simulink model "VCMGCM1962020b_v2"  (R2020b)
settings: Solver=FixedStepDiscrete  StartTime=0.0  StopTime=10.0  FixedStep=0.005  RelTol=1e-3  EnableMultiTasking=on
PreLoadFcn:
  | try, model_open; catch, disp('Error occurred while executing model pre-load callback: model_open.m'); disp('Please assure that the MATLAB working directory is set to the model directory before opening.'); end
InitFcn:
  | try, model_open; catch, end
undefined symbols (not defined in the file): Bridge, GCM, H, raptor_get_param_eval, raptor_get_safe_string, raptor_xcp_function
libraries: Blocks_lib x1165, Raptor_lib x665, simulink x62, VCM_lib x5
(part 17 of 23)

== system VCMGCM1962020b_v2/Fgnd/Control/Drive Inverter/Motor Torque Request/Inverter//Motor Limit & Request/Inverter Current Limit ==
  Split : Inport
  Bus Selector : BusSelector  OutputSignals=DrvInvtrMCLSplit [A],DrvInvtrGCLSplit [A]
  BusCreator : BusCreator  Inputs=2
  Header : Blocks_lib/Header  width=Portrait  addtext=''
  MinMax : MinMax  Inputs=2
  MinMax1 : MinMax  Inputs=2
  raptor_adjustment : Raptor_lib/Data Storage/raptor_adjustment  paramName=[invtrnam 'MCL']  nameSource=Parameter  initValue=0  dataType=double  storage=Calibration  calDispType=Number  calEnum={'Disabled', 'Enabled'}  calGain=1  calOffset=0  calMax=inf  calMin=-inf  calFormat=''  calUnit='A'  calHelp='Inverter motoring current limit'  calAccess=1  calFunction=group  calDispHeaders=off  calColHeaders={'Col1' 'Col2' 'Col3'}  calRowHeaders={'Row1' 'Row2' 'Row3'}
      settings: SourceProductName=Raptor
  raptor_adjustment1 : Raptor_lib/Data Storage/raptor_adjustment  paramName=[invtrnam 'GCL']  nameSource=Parameter  initValue=0  dataType=double  storage=Calibration  calDispType=Number  calEnum={'Disabled', 'Enabled'}  calGain=1  calOffset=0  calMax=inf  calMin=-inf  calFormat=''  calUnit='A'  calHelp='Inverter generating current limit'  calAccess=1  calFunction=group  calDispHeaders=off  calColHeaders={'Col1' 'Col2' 'Col3'}  calRowHeaders={'Row1' 'Row2' 'Row3'}
      settings: SourceProductName=Raptor
  InvtrCurLim : Outport  VectorParamsAs1DForOutWhenUnconnected=off
  wires:
  Bus Selector/1 -> MinMax/1  "<DrvInvtrMCLSplit [A]>"
  MinMax/1 -> BusCreator/1  "DrvInvtrMCL [A]"
  MinMax1/1 -> BusCreator/2  "DrvInvtrGCL [A]"
  BusCreator/1 -> InvtrCurLim/1  "InvtrCurLim"
  raptor_adjustment/1 -> MinMax/2
  raptor_adjustment1/1 -> MinMax1/2
  Split/1 -> Bus Selector/1
  Bus Selector/2 -> MinMax1/1  "<DrvInvtrGCLSplit [A]>"

== system VCMGCM1962020b_v2/Fgnd/Control/Drive Inverter/Motor Torque Request/Inverter//Motor Limit & Request/Motor Torque Limit ==
  Data : Inport
  EnblReq : Inport  Port=2
  InvtrCurLim : Inport  Port=3
  CAN : Subsystem
  Constant : Constant  Value=double([0 0])
  Current Control : Subsystem  mask{group=[group ' | Current Control']}
  Derate Multiplier : Subsystem
  Header : Blocks_lib/Header  width=Portrait  addtext=''
  Logical Operator : Logic  Operator=NOT  Inputs=1  AllPortsSameDT=off  OutDataTypeStr=boolean
  MinMax : MinMax  Inputs=3  InputSameDT=on
  MinMax1 : MinMax  Function=max  Inputs=3  InputSameDT=on
  Multiport Switch : MultiPortSwitch  DataPortOrder=Zero-based contiguous  Inputs=2  zeroidx=on
  Mux : Mux  Inputs=2
  Product : Product  InputSameDT=on  RndMeth=Zero  OutDataTypeStr=Inherit: Same as first input
  Product1 : Product  InputSameDT=on  RndMeth=Zero  OutDataTypeStr=Inherit: Same as first input
  Saturation : Saturate  UpperLimit=inf  LowerLimit=0
  Saturation1 : Saturate  UpperLimit=0  LowerLimit=-inf
  Selector : Selector  IndexMode=Zero-based  InputPortWidth=2  IndexOptions=Index vector (dialog)  Indices=[0]  OutputSizes=1
  Selector1 : Selector  IndexMode=Zero-based  InputPortWidth=2  IndexOptions=Index vector (dialog)  Indices=[0]  OutputSizes=1
  Selector2 : Selector  IndexMode=Zero-based  InputPortWidth=2  IndexOptions=Index vector (dialog)  Indices=[0]  OutputSizes=1
  Selector4 : Selector  IndexMode=Zero-based  InputPortWidth=2  IndexOptions=Index vector (dialog)  Indices=[1]  OutputSizes=1
  Selector5 : Selector  IndexMode=Zero-based  InputPortWidth=2  IndexOptions=Index vector (dialog)  Indices=[1]  OutputSizes=1
  Selector6 : Selector  IndexMode=Zero-based  InputPortWidth=2  IndexOptions=Index vector (dialog)  Indices=[1]  OutputSizes=1
  raptor_adjustment : Raptor_lib/Data Storage/raptor_adjustment  paramName=[mtrnam 'TrqLim_cal']  nameSource=Parameter  initValue=[0 0]  dataType=double  storage=Calibration  calDispType=Number  calEnum={}  calGain=1  calOffset=0  calMax=inf  calMin=-inf  calFormat=''  calUnit='Nm'  calHelp='Motor torque limit'  calAccess=1  calFunction=group  calDispHeaders=off  calColHeaders={'Col1' 'Col2' 'Col3'}  calRowHeaders={'Row1' 'Row2' 'Row3'}
      settings: SourceProductName=Raptor
  raptor_measurement : Raptor_lib/Data Storage/raptor_measurement  paramName=[mtrnam 'TrqLim']  nameSource=Parameter  calDispType=Number  calEnum={'Disabled', 'Enabled'}  calGain=1  calOffset=0  calMax=inf  calMin=-inf  calFormat=''  calUnit='Nm'  calHelp='Motor torque limit'  calAccess=1  calFunction=group  calVisible=on
      settings: SourceProductName=Raptor
  Nm : Outport  VectorParamsAs1DForOutWhenUnconnected=off
  wires:
  Product1/1 -> Saturation1/1
  Product/1 -> Saturation/1
  MinMax1/1 -> Product1/1
  MinMax/1 -> Product/1
  Saturation/1 -> Mux/1
  Saturation1/1 -> Mux/2
  Selector/1 -> MinMax/1
  Selector1/1 -> MinMax/2
  Selector2/1 -> MinMax/3
  Selector4/1 -> MinMax1/1
  Selector5/1 -> MinMax1/2
  Selector6/1 -> MinMax1/3
  Derate Multiplier/1(multp) -> Product1/2, Product/2
  CAN/1(Nm) -> Selector5/1, Selector1/1
  Current Control/1(Nm) -> Selector6/1, Selector2/1
  Data/1 -> CAN/1(Data), Current Control/1(Data), Derate Multiplier/1(Data)
  InvtrCurLim/1 -> Current Control/2(InvtrCurLim)
  EnblReq/1 -> Logical Operator/1
  Constant/1 -> Multiport Switch/3
  Mux/1 -> Multiport Switch/2
  Logical Operator/1 -> Multiport Switch/1
  Multiport Switch/1 -> Nm/1, raptor_measurement/1
  raptor_adjustment/1 -> Selector/1, Selector4/1

== system VCMGCM1962020b_v2/Fgnd/Control/Drive Inverter/Motor Torque Request/Inverter//Motor Limit & Request/Motor Torque Request ==
  note: Commenting this out. Won't require this logic with the new battery pack
  Data : Inport
  EnblReq : Inport  Port=2
  "Split " : Inport  Port=3
  TrqLim : Inport  Port=4
  Bus Selector : BusSelector  OutputSignals=DrvMtrTrqReqSplit [Nm]
  Bus Selector1 : BusSelector  Commented=on  OutputSignals=Sensors.CAN.Batt.HVES_Stress.Allowed_Discharge_Time.Allowed_Discharge_Time [s],Sensors.CAN.Batt.HVES_Stress.Allowed_Discharge_Time.Allowed_Discharge_TimeVld [Bool]
  Gain : Gain  Gain=-1  OutDataTypeStr=Inherit: Same as input
  Gearbox Preload : Subsystem
  Header : Blocks_lib/Header  width=Portrait  addtext=''
  Multiport Switch : MultiPortSwitch  DataPortOrder=Zero-based contiguous  Inputs=2  zeroidx=on
  Product : Product
  Rate Limit : Subsystem
      settings: PortSchema="{\"entries\":[{\"content\":{\"sides\":[{\"content\":{\"connectorIds\":[\"In1\",\"In2\"]},\"type\":\"ConnectorPlacement.EquallySpacedRectSide\",\"uuid\":\"af00f5e2-70f6-4d2c-ae48-24e87ed2ccff\"},{\"content\":{\"connectorIds\":[\"Out1\"],\"side\":\"RIGHT\"},\"type\":\"ConnectorPlacement.EquallySpacedRectSide\",\"uuid\":\"fb600a98-5a76-4cae-963e-f524cd2ffe01\"},{\"content\":{\"connectorIds\":[\"In3\"],\"side\":\"TOP\"},\"type\":\"ConnectorPlacement.EquallySpacedRectSide\",\"uuid\":\"705039ed-bc03-4a19-a3ef-f4fe93e8d60f\"},{\"content\":{\"connectorIds\":[],\"side\":\"HIDDEN\"},\"type\":\"ConnectorPlacement.EquallySpacedRectSide\",\"uuid\":\"fe928874-1757-472e-ae3f-ea99466837fe\"}]},\"type\":\"ConnectorPlacement.EquallySpacedConnector\",\"uuid\":\"90dd6add-1118-4843-b39b-045bdd8d2794\"}],\"packageUris\":[\"http://schema.mathworks.com/mf0/Connector/R2020b\"],\"version\":\"1.0\"}"
  Sat : Blocks_lib/Sat  SystemSampleTime=-1  VariantActivationTime=update diagram  Latency=0  AutoFrameSizeCalculation=off
  Switch : Switch  Commented=on  Criteria=u2 > Threshold
  Unit Delay : UnitDelay  SampleTime=-1  HasFrameUpgradeWarning=on
  raptor_adjustment : Raptor_lib/Data Storage/raptor_adjustment  paramName=[mtrnam 'TrqReqPolarity']  nameSource=Parameter  initValue=0  dataType=boolean  storage=Calibration  calDispType=Number  calEnum={'Disabled', 'Enabled'}  calGain=1  calOffset=0  calMax=inf  calMin=-inf  calFormat=''  calUnit='Bool'  calHelp='Motor torque request polarity (flip to change polarity)'  calAccess=1  calFunction=group  calDispHeaders=off  calColHeaders={'Col1' 'Col2' 'Col3'}  calRowHeaders={'Row1' 'Row2' 'Row3'}
      settings: SourceProductName=Raptor
  raptor_adjustment2 : Raptor_lib/Data Storage/raptor_adjustment  Commented=on  paramName='TrqLimDfltDrtMult'  nameSource=Parameter  initValue=1  dataType=double  storage=Calibration  calDispType=Number  calEnum={'Disabled', 'Enabled'}  calGain=1  calOffset=0  calMax=inf  calMin=-inf  calFormat=''  calUnit='Multiplier'  calHelp='Default derate multiplier on torque request based on '  calAccess=1  calFunction=group  calDispHeaders=off  calColHeaders={'Col1' 'Col2' 'Col3'}  calRowHeaders={'Row1' 'Row2' 'Row3'}
      settings: SourceProductName=Raptor
  raptor_table_1d : Raptor_lib/Table Lookup/raptor_table_1d  Commented=on  dataName='DischargeTimeMultplr'  initValue=[1,1,0,0]  dataType=double  storage=Calibration  initValueX=[20,15,10,5]  dataTypeXY=double  storageXY=Calibration  calVisible=on  showTable=on  calGain=1.0  calOffset=0.0  calMax=Inf  calMin=-Inf  calFormat='-1'  calUnit=''  calHelp=''  showBreakpoint=on  dataNameX=[]  calGainX=1.0  calOffsetX=0.0  calMaxX=Inf  calMinX=-Inf  calFormatX='-1'  calUnitX=''  calHelpX=''  calAccess=1  calFunction=group  measureEnable=on  mName=[raptor_get_param_eval(gcb,'dataName'), '_Output']
      settings: SourceProductName=Raptor
  Nm : Outport  VectorParamsAs1DForOutWhenUnconnected=off
  wires:
  TrqLim/1 -> Sat/2
  "Split "/1 -> Bus Selector/1
  Gain/1 -> Multiport Switch/3
  raptor_adjustment/1 -> Multiport Switch/1
  Bus Selector/1 -> Gearbox Preload/2(TrqReq)  "<DrvMtrTrqReqSplit [Nm]>"
  Data/1 -> Bus Selector1/1, Gearbox Preload/1(Data)
  EnblReq/1 -> Rate Limit/1(EnblReq)
  Gearbox Preload/1(Nm) -> Multiport Switch/2, Gain/1
  Rate Limit/1(Nm) -> Sat/1
  Sat/1 -> Unit Delay/1, Nm/1
  Unit Delay/1 -> Rate Limit/2(TrqReq1/z)
  raptor_adjustment2/1 -> Switch/3
  raptor_table_1d/1 -> Switch/1
  Bus Selector1/2 -> Switch/2  "<Allowed_Discharge_TimeVld [Bool]>"
  Bus Selector1/1 -> raptor_table_1d/1  "<Allowed_Discharge_Time [s]>"
  Switch/1 -> Product/2
  Multiport Switch/1 -> Product/1
  Product/1 -> Rate Limit/3(TrqReq)

== system VCMGCM1962020b_v2/Fgnd/Control/Modes/Startup & Shutdown/HV System Disable/Flash Started ==
  note: Note:
      | Raptor-Cal transmits the 0x7DF UDS message before starting to flash the GCM196.
      | This code is not relevant for other modules.
  Header : Blocks_lib/Header  width=Portrait  addtext=''
  Terminator{,1..4} (5 alike) : Terminator
  UDS Msg Rxd : Subsystem
  raptor_can_rxraw : Raptor_lib/CAN/raptor_can_rxraw  canBus='CAN1'  extendedId=0  showAge=1  id=hex2dec('7DF')  idMask=hex2dec('7FF')  mailbox='UDSMsg'  queueSize=1
      settings: SourceProductName=Raptor
  raptor_can_trigger : Raptor_lib/CAN/raptor_can_trigger  mailbox='UDSMsg'  inherited=1  alwaysEnabled=1  triggerPriority=0
      settings: SourceProductName=Raptor
  raptor_data_read : Raptor_lib/Data Storage/raptor_data_read  dataName='VCMFlashStarted'  dataShape=Scalar  idxSource=Input  idxRow=1  idxCol=1
      settings: SourceProductName=Raptor
  Bool : Outport  VectorParamsAs1DForOutWhenUnconnected=off
  wires:
  raptor_can_rxraw/1 -> Terminator/1
  raptor_can_rxraw/2 -> Terminator1/1
  raptor_can_rxraw/4 -> Terminator3/1
  raptor_can_rxraw/3 -> Terminator2/1
  raptor_can_rxraw/5 -> Terminator4/1
  raptor_can_trigger/1 -> UDS Msg Rxd/Trigger
  raptor_data_read/1 -> Bool/1

== system VCMGCM1962020b_v2/Fgnd/Control/Modes/Startup & Shutdown/HV System Disable/HVSysDsblLevel1 ==
  Data : Inport
  Bus Selector : BusSelector  OutputSignals=VirtualSensors.Spd.VehSpd [kph]
  Header : Blocks_lib/Header  width=Portrait  addtext=''
  Logical Operator : Logic  OutDataTypeStr=boolean
  Logical Operator1 : Logic  Operator=NOT  OutDataTypeStr=boolean
  Relational Operator : RelationalOperator  Operator=<=  OutDataTypeStr=boolean  RndMeth=Nearest
  SetRst : Blocks_lib/SetRst  init=0
  raptor_adjustment : Raptor_lib/Data Storage/raptor_adjustment  paramName='HVSysDsblLevel1VehSpdMx'  nameSource=Parameter  initValue=0  dataType=double  storage=Calibration  calDispType=Number  calEnum={'False', 'True'}  calGain=1  calOffset=0.0  calMax=inf  calMin=-inf  calFormat=''  calUnit='kph'  calHelp='High-voltage system disable (level 1) vehicle speed maximum'  calAccess=1  calFunction=group  calDispHeaders=off  calColHeaders={'Col1' 'Col2' 'Col3'}  calRowHeaders={'Row1' 'Row2' 'Row3'}
      settings: SourceProductName=Raptor
  raptor_fault_action : Raptor_lib/Faults/raptor_fault_action  actionName='HVSysDsblLevel1'  calVisible=off  calAccess=1  calFunction='System | FaultManager | FaultAction'
      settings: SourceProductName=Raptor
  Bool : Outport  VectorParamsAs1DForOutWhenUnconnected=off
  wires:
  Data/1 -> Bus Selector/1
  SetRst/1 -> Bool/1
  Relational Operator/1 -> Logical Operator/2
  raptor_adjustment/1 -> Relational Operator/2
  Bus Selector/1 -> Relational Operator/1  "<VehSpd [kph]>"
  Logical Operator/1 -> SetRst/1
  Logical Operator1/1 -> SetRst/2
  raptor_fault_action/1 -> Logical Operator/1, Logical Operator1/1

== system VCMGCM1962020b_v2/Fgnd/Control/Modes/Startup & Shutdown/HV System Disable/Not Run Mode or Charge Plug Disconnected ==
  Data : Inport
  AND : Logic  Inputs=3  AllPortsSameDT=off  OutDataTypeStr=boolean
  Bus Selector1 : BusSelector  OutputSignals=Control.Mode.StartStop.RunMode [Bool],Sensors.Sensors.Volt.WakeChgr.WakeChgrVld [Bool],Sensors.Sensors.Volt.WakeChgr.WakeChgr [Bool]
  Header : Blocks_lib/Header  width=Portrait  addtext=''
  Unit Delay : UnitDelay  SampleTime=-1  HasFrameUpgradeWarning=on
  Bool : Outport  VectorParamsAs1DForOutWhenUnconnected=off
  wires:
  Data/1 -> Bus Selector1/1
  Bus Selector1/1 -> Unit Delay/1  "<RunMode [Bool]>"
  AND/1 -> Bool/1
  Unit Delay/1 -> AND/1
  Bus Selector1/3 -> AND/3  "<WakeChgr [Bool]>"
  Bus Selector1/2 -> AND/2  "<WakeChgrVld [Bool]>"

== system VCMGCM1962020b_v2/Fgnd/Control/Modes/Startup & Shutdown/HV System Disable/Wait to Disable ==
  Data : Inport
  Abs : Abs
  Bus Selector : BusSelector  OutputSignals=VirtualSensors.DrvInvtr.DrvMtrSpd [rpm]
  Header : Blocks_lib/Header  width=Portrait  addtext=''
  Relational Operator : RelationalOperator  OutDataTypeStr=boolean  RndMeth=Nearest
  raptor_adjustment : Raptor_lib/Data Storage/raptor_adjustment  paramName='HVSysDsblDrvMtrSpdMx'  nameSource=Parameter  initValue=0  dataType=double  storage=Calibration  calDispType=Number  calEnum={'False', 'True'}  calGain=1  calOffset=0.0  calMax=inf  calMin=-inf  calFormat=''  calUnit='rpm'  calHelp='High-voltage system disable drive motor speed maximum'  calAccess=1  calFunction=group  calDispHeaders=off  calColHeaders={'Col1' 'Col2' 'Col3'}  calRowHeaders={'Row1' 'Row2' 'Row3'}
      settings: SourceProductName=Raptor
  Bool : Outport  VectorParamsAs1DForOutWhenUnconnected=off
  wires:
  Data/1 -> Bus Selector/1
  Relational Operator/1 -> Bool/1
  raptor_adjustment/1 -> Relational Operator/2
  Bus Selector/1 -> Abs/1  "<DrvMtrSpd [rpm]>"
  Abs/1 -> Relational Operator/1

== system VCMGCM1962020b_v2/Fgnd/Diagnostics/Diagnostics/CAN Bus Passive/EvalDiag/CAN1 ==
  CmprToBit : Blocks_lib/CmprToBit  op===  val=2048  enum={'Disabled', 'Enabled'}
  FltTmr : Blocks_lib/FltTmr  nam=[bus 'BusPassive']  tmrth_nam=[bus 'BusPassiveTimeThr']  tmrth_typ=uint16  tmrth_help='CAN bus passive fault time threshold'  samptime=samptime  group='Diagnostics | CAN'
  Header : Blocks_lib/Header  width=Portrait  addtext=''
  raptor_can_state : Raptor_lib/CAN/raptor_can_state  resourceValues=CAN1|CAN2|CAN3|(None)  resource=CAN1  errOut='RAPTOR MASK DEFAULT'
      settings: SourceProductName=Raptor
  raptor_can_tx_queue_info : Raptor_lib/CAN/raptor_can_tx_queue_info  resourceValues=CAN1|CAN2|CAN3|(None)  resource=CAN1  queueValues=Receive|Transmit  queue=Receive
      settings: SourceProductName=Raptor
  raptor_can_tx_queue_info1 : Raptor_lib/CAN/raptor_can_tx_queue_info  resourceValues=CAN1|CAN2|CAN3|(None)  resource=CAN1  queueValues=Receive|Transmit  queue=Transmit
      settings: SourceProductName=Raptor
  raptor_measurement : Raptor_lib/Data Storage/raptor_measurement  paramName=[bus 'State']  nameSource=Parameter  calDispType=Number  calEnum={}  calGain=1.0  calOffset=0.0  calMax=inf  calMin=-inf  calFormat='-1'  calUnit='bitfield'  calHelp='CAN state'  calAccess=1  calFunction='Diagnostics | CAN'  calVisible=on
      settings: SourceProductName=Raptor
  raptor_measurement1 : Raptor_lib/Data Storage/raptor_measurement  paramName=[bus 'RxErrCount']  nameSource=Parameter  calDispType=Number  calEnum={'False', 'True'}  calGain=1.0  calOffset=0.0  calMax=inf  calMin=-inf  calFormat='-1'  calUnit='count'  calHelp='CAN Rx error count'  calAccess=1  calFunction='Diagnostics | CAN'  calVisible=on
      settings: SourceProductName=Raptor
  raptor_measurement10 : Raptor_lib/Data Storage/raptor_measurement  paramName=[bus 'TxQueueOverruns']  nameSource=Parameter  calDispType=Number  calEnum={'False', 'True'}  calGain=1.0  calOffset=0.0  calMax=inf  calMin=-inf  calFormat='-1'  calUnit='count'  calHelp='CAN Tx queue overruns'  calAccess=1  calFunction='Diagnostics | CAN'  calVisible=on
      settings: SourceProductName=Raptor
  raptor_measurement2 : Raptor_lib/Data Storage/raptor_measurement  paramName=[bus 'TxErrCount']  nameSource=Parameter  calDispType=Number  calEnum={'False', 'True'}  calGain=1.0  calOffset=0.0  calMax=inf  calMin=-inf  calFormat='-1'  calUnit='count'  calHelp='CAN Tx error count'  calAccess=1  calFunction='Diagnostics | CAN'  calVisible=on
      settings: SourceProductName=Raptor
  raptor_measurement3 : Raptor_lib/Data Storage/raptor_measurement  paramName=[bus 'RxQueueSize']  nameSource=Parameter  calDispType=Number  calEnum={'False', 'True'}  calGain=1.0  calOffset=0.0  calMax=inf  calMin=-inf  calFormat='-1'  calUnit='count'  calHelp='CAN Rx queue size'  calAccess=1  calFunction='Diagnostics | CAN'  calVisible=on
      settings: SourceProductName=Raptor
  raptor_measurement4 : Raptor_lib/Data Storage/raptor_measurement  paramName=[bus 'RxQueueDepth']  nameSource=Parameter  calDispType=Number  calEnum={'False', 'True'}  calGain=1.0  calOffset=0.0  calMax=inf  calMin=-inf  calFormat='-1'  calUnit='count'  calHelp='CAN Rx queue depth'  calAccess=1  calFunction='Diagnostics | CAN'  calVisible=on
      settings: SourceProductName=Raptor
  raptor_measurement5 : Raptor_lib/Data Storage/raptor_measurement  paramName=[bus 'RxQueueMaxDepth']  nameSource=Parameter  calDispType=Number  calEnum={'False', 'True'}  calGain=1.0  calOffset=0.0  calMax=inf  calMin=-inf  calFormat='-1'  calUnit='count'  calHelp='CAN Rx queue maximum depth'  calAccess=1  calFunction='Diagnostics | CAN'  calVisible=on
      settings: SourceProductName=Raptor
  raptor_measurement6 : Raptor_lib/Data Storage/raptor_measurement  paramName=[bus 'RxQueueOverruns']  nameSource=Parameter  calDispType=Number  calEnum={'False', 'True'}  calGain=1.0  calOffset=0.0  calMax=inf  calMin=-inf  calFormat='-1'  calUnit='count'  calHelp='CAN Rx queue overruns'  calAccess=1  calFunction='Diagnostics | CAN'  calVisible=on
      settings: SourceProductName=Raptor
  raptor_measurement7 : Raptor_lib/Data Storage/raptor_measurement  paramName=[bus 'TxQueueSize']  nameSource=Parameter  calDispType=Number  calEnum={'False', 'True'}  calGain=1.0  calOffset=0.0  calMax=inf  calMin=-inf  calFormat='-1'  calUnit='count'  calHelp='CAN Tx queue size'  calAccess=1  calFunction='Diagnostics | CAN'  calVisible=on
      settings: SourceProductName=Raptor
  raptor_measurement8 : Raptor_lib/Data Storage/raptor_measurement  paramName=[bus 'TxQueueDepth']  nameSource=Parameter  calDispType=Number  calEnum={'False', 'True'}  calGain=1.0  calOffset=0.0  calMax=inf  calMin=-inf  calFormat='-1'  calUnit='count'  calHelp='CAN Tx queue depth'  calAccess=1  calFunction='Diagnostics | CAN'  calVisible=on
      settings: SourceProductName=Raptor
  raptor_measurement9 : Raptor_lib/Data Storage/raptor_measurement  paramName=[bus 'TxQueueMaxDepth']  nameSource=Parameter  calDispType=Number  calEnum={'False', 'True'}  calGain=1.0  calOffset=0.0  calMax=inf  calMin=-inf  calFormat='-1'  calUnit='count'  calHelp='CAN Tx queue maximum depth'  calAccess=1  calFunction='Diagnostics | CAN'  calVisible=on
      settings: SourceProductName=Raptor
  wires:
  CmprToBit/1 -> FltTmr/1
  raptor_can_state/2 -> raptor_measurement1/1
  raptor_can_state/1 -> raptor_measurement/1, CmprToBit/1
  raptor_can_state/3 -> raptor_measurement2/1
  raptor_can_tx_queue_info/1 -> raptor_measurement3/1
  raptor_can_tx_queue_info/2 -> raptor_measurement4/1
  raptor_can_tx_queue_info/3 -> raptor_measurement5/1
  raptor_can_tx_queue_info/4 -> raptor_measurement6/1
  raptor_can_tx_queue_info1/1 -> raptor_measurement7/1
  raptor_can_tx_queue_info1/3 -> raptor_measurement9/1
  raptor_can_tx_queue_info1/4 -> raptor_measurement10/1
  raptor_can_tx_queue_info1/2 -> raptor_measurement8/1

== system VCMGCM1962020b_v2/Fgnd/Diagnostics/Diagnostics/CAN Bus Passive/EvalDiag/CAN2 ==
  CmprToBit : Blocks_lib/CmprToBit  op===  val=2048  enum={'Disabled', 'Enabled'}
  FltTmr : Blocks_lib/FltTmr  nam=[bus 'BusPassive']  tmrth_nam=[bus 'BusPassiveTimeThr']  tmrth_typ=uint16  tmrth_help='CAN bus passive fault time threshold'  samptime=samptime  group='Diagnostics | CAN'
  Header : Blocks_lib/Header  width=Portrait  addtext=''
  raptor_can_state : Raptor_lib/CAN/raptor_can_state  resourceValues=CAN1|CAN2|CAN3|(None)  resource=CAN2  errOut='RAPTOR MASK DEFAULT'
      settings: SourceProductName=Raptor
  raptor_can_tx_queue_info : Raptor_lib/CAN/raptor_can_tx_queue_info  resourceValues=CAN1|CAN2|CAN3|(None)  resource=CAN2  queueValues=Receive|Transmit  queue=Receive
      settings: SourceProductName=Raptor
  raptor_can_tx_queue_info1 : Raptor_lib/CAN/raptor_can_tx_queue_info  resourceValues=CAN1|CAN2|CAN3|(None)  resource=CAN2  queueValues=Receive|Transmit  queue=Transmit
      settings: SourceProductName=Raptor
  raptor_measurement : Raptor_lib/Data Storage/raptor_measurement  paramName=[bus 'State']  nameSource=Parameter  calDispType=Number  calEnum={}  calGain=1.0  calOffset=0.0  calMax=inf  calMin=-inf  calFormat='-1'  calUnit='bitfield'  calHelp='CAN state'  calAccess=1  calFunction='Diagnostics | CAN'  calVisible=on
      settings: SourceProductName=Raptor
  raptor_measurement1 : Raptor_lib/Data Storage/raptor_measurement  paramName=[bus 'RxErrCount']  nameSource=Parameter  calDispType=Number  calEnum={'False', 'True'}  calGain=1.0  calOffset=0.0  calMax=inf  calMin=-inf  calFormat='-1'  calUnit='count'  calHelp='CAN Rx error count'  calAccess=1  calFunction='Diagnostics | CAN'  calVisible=on
      settings: SourceProductName=Raptor
  raptor_measurement10 : Raptor_lib/Data Storage/raptor_measurement  paramName=[bus 'TxQueueOverruns']  nameSource=Parameter  calDispType=Number  calEnum={'False', 'True'}  calGain=1.0  calOffset=0.0  calMax=inf  calMin=-inf  calFormat='-1'  calUnit='count'  calHelp='CAN Tx queue overruns'  calAccess=1  calFunction='Diagnostics | CAN'  calVisible=on
      settings: SourceProductName=Raptor
  raptor_measurement2 : Raptor_lib/Data Storage/raptor_measurement  paramName=[bus 'TxErrCount']  nameSource=Parameter  calDispType=Number  calEnum={'False', 'True'}  calGain=1.0  calOffset=0.0  calMax=inf  calMin=-inf  calFormat='-1'  calUnit='count'  calHelp='CAN Tx error count'  calAccess=1  calFunction='Diagnostics | CAN'  calVisible=on
      settings: SourceProductName=Raptor
  raptor_measurement3 : Raptor_lib/Data Storage/raptor_measurement  paramName=[bus 'RxQueueSize']  nameSource=Parameter  calDispType=Number  calEnum={'False', 'True'}  calGain=1.0  calOffset=0.0  calMax=inf  calMin=-inf  calFormat='-1'  calUnit='count'  calHelp='CAN Rx queue size'  calAccess=1  calFunction='Diagnostics | CAN'  calVisible=on
      settings: SourceProductName=Raptor
  raptor_measurement4 : Raptor_lib/Data Storage/raptor_measurement  paramName=[bus 'RxQueueDepth']  nameSource=Parameter  calDispType=Number  calEnum={'False', 'True'}  calGain=1.0  calOffset=0.0  calMax=inf  calMin=-inf  calFormat='-1'  calUnit='count'  calHelp='CAN Rx queue depth'  calAccess=1  calFunction='Diagnostics | CAN'  calVisible=on
      settings: SourceProductName=Raptor
  raptor_measurement5 : Raptor_lib/Data Storage/raptor_measurement  paramName=[bus 'RxQueueMaxDepth']  nameSource=Parameter  calDispType=Number  calEnum={'False', 'True'}  calGain=1.0  calOffset=0.0  calMax=inf  calMin=-inf  calFormat='-1'  calUnit='count'  calHelp='CAN Rx queue maximum depth'  calAccess=1  calFunction='Diagnostics | CAN'  calVisible=on
      settings: SourceProductName=Raptor
  raptor_measurement6 : Raptor_lib/Data Storage/raptor_measurement  paramName=[bus 'RxQueueOverruns']  nameSource=Parameter  calDispType=Number  calEnum={'False', 'True'}  calGain=1.0  calOffset=0.0  calMax=inf  calMin=-inf  calFormat='-1'  calUnit='count'  calHelp='CAN Rx queue overruns'  calAccess=1  calFunction='Diagnostics | CAN'  calVisible=on
      settings: SourceProductName=Raptor
  raptor_measurement7 : Raptor_lib/Data Storage/raptor_measurement  paramName=[bus 'TxQueueSize']  nameSource=Parameter  calDispType=Number  calEnum={'False', 'True'}  calGain=1.0  calOffset=0.0  calMax=inf  calMin=-inf  calFormat='-1'  calUnit='count'  calHelp='CAN Tx queue size'  calAccess=1  calFunction='Diagnostics | CAN'  calVisible=on
      settings: SourceProductName=Raptor
  raptor_measurement8 : Raptor_lib/Data Storage/raptor_measurement  paramName=[bus 'TxQueueDepth']  nameSource=Parameter  calDispType=Number  calEnum={'False', 'True'}  calGain=1.0  calOffset=0.0  calMax=inf  calMin=-inf  calFormat='-1'  calUnit='count'  calHelp='CAN Tx queue depth'  calAccess=1  calFunction='Diagnostics | CAN'  calVisible=on
      settings: SourceProductName=Raptor
  raptor_measurement9 : Raptor_lib/Data Storage/raptor_measurement  paramName=[bus 'TxQueueMaxDepth']  nameSource=Parameter  calDispType=Number  calEnum={'False', 'True'}  calGain=1.0  calOffset=0.0  calMax=inf  calMin=-inf  calFormat='-1'  calUnit='count'  calHelp='CAN Tx queue maximum depth'  calAccess=1  calFunction='Diagnostics | CAN'  calVisible=on
      settings: SourceProductName=Raptor
  wires:
  raptor_can_tx_queue_info1/2 -> raptor_measurement8/1
  raptor_can_tx_queue_info1/4 -> raptor_measurement10/1
  raptor_can_tx_queue_info1/3 -> raptor_measurement9/1
  raptor_can_tx_queue_info1/1 -> raptor_measurement7/1
  raptor_can_tx_queue_info/4 -> raptor_measurement6/1
  raptor_can_tx_queue_info/3 -> raptor_measurement5/1
  raptor_can_tx_queue_info/2 -> raptor_measurement4/1
  raptor_can_tx_queue_info/1 -> raptor_measurement3/1
  raptor_can_state/3 -> raptor_measurement2/1
  raptor_can_state/1 -> CmprToBit/1, raptor_measurement/1
  raptor_can_state/2 -> raptor_measurement1/1
  CmprToBit/1 -> FltTmr/1

== system VCMGCM1962020b_v2/Fgnd/Diagnostics/Diagnostics/CAN Bus Passive/EvalDiag/CAN3 ==
  CmprToBit : Blocks_lib/CmprToBit  op===  val=2048  enum={'Disabled', 'Enabled'}
  FltTmr : Blocks_lib/FltTmr  nam=[bus 'BusPassive']  tmrth_nam=[bus 'BusPassiveTimeThr']  tmrth_typ=uint16  tmrth_help='CAN bus passive fault time threshold'  samptime=samptime  group='Diagnostics | CAN'
  Header : Blocks_lib/Header  width=Portrait  addtext=''
  raptor_can_state : Raptor_lib/CAN/raptor_can_state  resourceValues=CAN1|CAN2|CAN3|(None)  resource=CAN3  errOut='RAPTOR MASK DEFAULT'
      settings: SourceProductName=Raptor
  raptor_can_tx_queue_info : Raptor_lib/CAN/raptor_can_tx_queue_info  resourceValues=CAN1|CAN2|CAN3|(None)  resource=CAN3  queueValues=Receive|Transmit  queue=Receive
      settings: SourceProductName=Raptor
  raptor_can_tx_queue_info1 : Raptor_lib/CAN/raptor_can_tx_queue_info  resourceValues=CAN1|CAN2|CAN3|(None)  resource=CAN3  queueValues=Receive|Transmit  queue=Transmit
      settings: SourceProductName=Raptor
  raptor_measurement : Raptor_lib/Data Storage/raptor_measurement  paramName=[bus 'State']  nameSource=Parameter  calDispType=Number  calEnum={}  calGain=1.0  calOffset=0.0  calMax=inf  calMin=-inf  calFormat='-1'  calUnit='bitfield'  calHelp='CAN state'  calAccess=1  calFunction='Diagnostics | CAN'  calVisible=on
      settings: SourceProductName=Raptor
  raptor_measurement1 : Raptor_lib/Data Storage/raptor_measurement  paramName=[bus 'RxErrCount']  nameSource=Parameter  calDispType=Number  calEnum={'False', 'True'}  calGain=1.0  calOffset=0.0  calMax=inf  calMin=-inf  calFormat='-1'  calUnit='count'  calHelp='CAN Rx error count'  calAccess=1  calFunction='Diagnostics | CAN'  calVisible=on
      settings: SourceProductName=Raptor
  raptor_measurement10 : Raptor_lib/Data Storage/raptor_measurement  paramName=[bus 'TxQueueOverruns']  nameSource=Parameter  calDispType=Number  calEnum={'False', 'True'}  calGain=1.0  calOffset=0.0  calMax=inf  calMin=-inf  calFormat='-1'  calUnit='count'  calHelp='CAN Tx queue overruns'  calAccess=1  calFunction='Diagnostics | CAN'  calVisible=on
      settings: SourceProductName=Raptor
  raptor_measurement2 : Raptor_lib/Data Storage/raptor_measurement  paramName=[bus 'TxErrCount']  nameSource=Parameter  calDispType=Number  calEnum={'False', 'True'}  calGain=1.0  calOffset=0.0  calMax=inf  calMin=-inf  calFormat='-1'  calUnit='count'  calHelp='CAN Tx error count'  calAccess=1  calFunction='Diagnostics | CAN'  calVisible=on
      settings: SourceProductName=Raptor
  raptor_measurement3 : Raptor_lib/Data Storage/raptor_measurement  paramName=[bus 'RxQueueSize']  nameSource=Parameter  calDispType=Number  calEnum={'False', 'True'}  calGain=1.0  calOffset=0.0  calMax=inf  calMin=-inf  calFormat='-1'  calUnit='count'  calHelp='CAN Rx queue size'  calAccess=1  calFunction='Diagnostics | CAN'  calVisible=on
      settings: SourceProductName=Raptor
  raptor_measurement4 : Raptor_lib/Data Storage/raptor_measurement  paramName=[bus 'RxQueueDepth']  nameSource=Parameter  calDispType=Number  calEnum={'False', 'True'}  calGain=1.0  calOffset=0.0  calMax=inf  calMin=-inf  calFormat='-1'  calUnit='count'  calHelp='CAN Rx queue depth'  calAccess=1  calFunction='Diagnostics | CAN'  calVisible=on
      settings: SourceProductName=Raptor
  raptor_measurement5 : Raptor_lib/Data Storage/raptor_measurement  paramName=[bus 'RxQueueMaxDepth']  nameSource=Parameter  calDispType=Number  calEnum={'False', 'True'}  calGain=1.0  calOffset=0.0  calMax=inf  calMin=-inf  calFormat='-1'  calUnit='count'  calHelp='CAN Rx queue maximum depth'  calAccess=1  calFunction='Diagnostics | CAN'  calVisible=on
      settings: SourceProductName=Raptor
  raptor_measurement6 : Raptor_lib/Data Storage/raptor_measurement  paramName=[bus 'RxQueueOverruns']  nameSource=Parameter  calDispType=Number  calEnum={'False', 'True'}  calGain=1.0  calOffset=0.0  calMax=inf  calMin=-inf  calFormat='-1'  calUnit='count'  calHelp='CAN Rx queue overruns'  calAccess=1  calFunction='Diagnostics | CAN'  calVisible=on
      settings: SourceProductName=Raptor
  raptor_measurement7 : Raptor_lib/Data Storage/raptor_measurement  paramName=[bus 'TxQueueSize']  nameSource=Parameter  calDispType=Number  calEnum={'False', 'True'}  calGain=1.0  calOffset=0.0  calMax=inf  calMin=-inf  calFormat='-1'  calUnit='count'  calHelp='CAN Tx queue size'  calAccess=1  calFunction='Diagnostics | CAN'  calVisible=on
      settings: SourceProductName=Raptor
  raptor_measurement8 : Raptor_lib/Data Storage/raptor_measurement  paramName=[bus 'TxQueueDepth']  nameSource=Parameter  calDispType=Number  calEnum={'False', 'True'}  calGain=1.0  calOffset=0.0  calMax=inf  calMin=-inf  calFormat='-1'  calUnit='count'  calHelp='CAN Tx queue depth'  calAccess=1  calFunction='Diagnostics | CAN'  calVisible=on
      settings: SourceProductName=Raptor
  raptor_measurement9 : Raptor_lib/Data Storage/raptor_measurement  paramName=[bus 'TxQueueMaxDepth']  nameSource=Parameter  calDispType=Number  calEnum={'False', 'True'}  calGain=1.0  calOffset=0.0  calMax=inf  calMin=-inf  calFormat='-1'  calUnit='count'  calHelp='CAN Tx queue maximum depth'  calAccess=1  calFunction='Diagnostics | CAN'  calVisible=on
      settings: SourceProductName=Raptor
  wires:
  CmprToBit/1 -> FltTmr/1
  raptor_can_state/2 -> raptor_measurement1/1
  raptor_can_state/1 -> raptor_measurement/1, CmprToBit/1
  raptor_can_state/3 -> raptor_measurement2/1
  raptor_can_tx_queue_info/1 -> raptor_measurement3/1
  raptor_can_tx_queue_info/2 -> raptor_measurement4/1
  raptor_can_tx_queue_info/3 -> raptor_measurement5/1
  raptor_can_tx_queue_info/4 -> raptor_measurement6/1
  raptor_can_tx_queue_info1/1 -> raptor_measurement7/1
  raptor_can_tx_queue_info1/3 -> raptor_measurement9/1
  raptor_can_tx_queue_info1/4 -> raptor_measurement10/1
  raptor_can_tx_queue_info1/2 -> raptor_measurement8/1

== system VCMGCM1962020b_v2/Fgnd/Diagnostics/Diagnostics/HVIL X-Check/EvalDiag/HVIL X-Check/EvalDiag ==
  Status : Inport
  f : TriggerPort  TriggerType=function-call  VariantControl=(inherit)
      settings: CopyFcn=Stateflow.SLINSF.SimulinkMan.removeBlockPreDeleteFcn  PreDeleteFcn=Stateflow.SLINSF.SimulinkMan.unsafePredeleteFcn
  Header : Blocks_lib/Header  width=Portrait  addtext=''
  raptor_fault_def : Raptor_lib/Faults/raptor_fault_def  faultName='HVILXChk'  persist=off  sticky=off  emisRelated=off  singleTrip=off  clearMethod=Standard  xLimit=1  yLimit=1  calEnable=on  addDisable=off  calAccess=1  calFunction=['Diagnostics | Fault Defs | ' raptor_get_param_eval(gcb, 'faultName')]
      settings: SourceProductName=Raptor
  wires:
  Status/1 -> raptor_fault_def/1

== system VCMGCM1962020b_v2/Fgnd/Diagnostics/Fault Statuses/Status Marquees/Display first 7 faults with the selected state1/Cycle Through Remaining Faults ==
  NumOfFltsTotal : Inport
  IdxOfLastFltToSkip : Inport  Port=2
  NumOfFltsToSkip : Inport  Port=3
  Header : Blocks_lib/Header  width=Portrait  addtext=''
  Increment Stored Integer5 : simulink/Additional Math & Discrete/Additional Math: Increment - Decrement/Increment Stored Integer
  MinMax : MinMax  Function=max  Inputs=2
  Multiport Switch7 : MultiPortSwitch  DataPortOrder=Zero-based contiguous  Inputs=2  zeroidx=on
  Relational Operator7 : RelationalOperator  Operator=<  OutDataTypeStr=boolean  RndMeth=Nearest
  Unit Delay : UnitDelay  SampleTime=-1  HasFrameUpgradeWarning=on
  raptor_fault_measurement5 : Raptor_lib/Faults/raptor_fault_measurement  dataName=[finalVarName 'Loop']  calHelp='one of the faults that have failed this drive cycle'  calAccess=1  calFunction=[group ' | ' finalVarName]
      settings: SourceProductName=Raptor
  raptor_fault_null8 : Raptor_lib/Faults/raptor_fault_null  null=0
      settings: SourceProductName=Raptor
  raptor_fault_stateIterator6 : Raptor_lib/Faults/raptor_fault_stateIterator  notOccurred=off  suspected=off  active=off  occurred=off  failedThisDC=off  testCmpltThisDC=off  failing=on  pending=off  confirmed=off  mil=off  permanent=off  ready=off  prevConfirmed=off  failedSinceClear=off  failedLastDC=off  prevMil=off
      settings: SourceProductName=Raptor
  wires:
  NumOfFltsToSkip/1 -> Increment Stored Integer5/1
  IdxOfLastFltToSkip/1 -> MinMax/1
  NumOfFltsTotal/1 -> Relational Operator7/1
  Unit Delay/1 -> MinMax/2
  Multiport Switch7/1 -> raptor_fault_measurement5/1
  raptor_fault_stateIterator6/1 -> Multiport Switch7/2, Unit Delay/1
  Relational Operator7/1 -> Multiport Switch7/1
  raptor_fault_null8/1 -> Multiport Switch7/3
  Increment Stored Integer5/1 -> Relational Operator7/2
  MinMax/1 -> raptor_fault_stateIterator6/1

== system VCMGCM1962020b_v2/Fgnd/Diagnostics/Fault Statuses/Status Marquees/Display first 7 faults with the selected state2/Cycle Through Remaining Faults ==
  NumOfFltsTotal : Inport
  IdxOfLastFltToSkip : Inport  Port=2
  NumOfFltsToSkip : Inport  Port=3
  Header : Blocks_lib/Header  width=Portrait  addtext=''
  Increment Stored Integer5 : simulink/Additional Math & Discrete/Additional Math: Increment - Decrement/Increment Stored Integer
  MinMax : MinMax  Function=max  Inputs=2
  Multiport Switch7 : MultiPortSwitch  DataPortOrder=Zero-based contiguous  Inputs=2  zeroidx=on
  Relational Operator7 : RelationalOperator  Operator=<  OutDataTypeStr=boolean  RndMeth=Nearest
  Unit Delay : UnitDelay  SampleTime=-1  HasFrameUpgradeWarning=on
  raptor_fault_measurement5 : Raptor_lib/Faults/raptor_fault_measurement  dataName=[finalVarName 'Loop']  calHelp='one of the faults that have failed this drive cycle'  calAccess=1  calFunction=[group ' | ' finalVarName]
      settings: SourceProductName=Raptor
  raptor_fault_null8 : Raptor_lib/Faults/raptor_fault_null  null=0
      settings: SourceProductName=Raptor
  raptor_fault_stateIterator6 : Raptor_lib/Faults/raptor_fault_stateIterator  notOccurred=off  suspected=off  active=off  occurred=off  failedThisDC=on  testCmpltThisDC=off  failing=off  pending=off  confirmed=off  mil=off  permanent=off  ready=off  prevConfirmed=off  failedSinceClear=off  failedLastDC=off  prevMil=off
      settings: SourceProductName=Raptor
  wires:
  MinMax/1 -> raptor_fault_stateIterator6/1
  Increment Stored Integer5/1 -> Relational Operator7/2
  raptor_fault_null8/1 -> Multiport Switch7/3
  Relational Operator7/1 -> Multiport Switch7/1
  raptor_fault_stateIterator6/1 -> Unit Delay/1, Multiport Switch7/2
  Multiport Switch7/1 -> raptor_fault_measurement5/1
  Unit Delay/1 -> MinMax/2
  NumOfFltsTotal/1 -> Relational Operator7/1
  IdxOfLastFltToSkip/1 -> MinMax/1
  NumOfFltsToSkip/1 -> Increment Stored Integer5/1

== system VCMGCM1962020b_v2/Fgnd/Sensors/CAN/Inverter/EM2_InvTemp/EM2InvTemp ==
  DiagEnbl : Inport
  Enable : EnablePort
  CANRxFieldSingleFloat : Subsystem  AncestorBlock=Blocks_lib/CANRxField  mask(CANRxField){typ='double', custom=off, custom_nam='---', custom_units='---'}
      mask prompts: typ "Field Data Type"; custom "Use Custom Name and Units (instead of from .dbc file)"; custom_nam "Custom Name"; custom_units "Custom Units"
      mask help:
      | To be used with the raptor_can_rxmsg block.
      |
      | By default, the field name/units will be inherited from the .dbc file. For Custom Name or Units, check the checkbox. To use the inherited name/units in the custom name/units, use the string '---' to inhereit. For example, to simply add a prefix, the custom name would be something like 'prefix_---'.
      mask init:
      | cb = gcb;
      | 
      | % --- Find Message Name
      | par = get_param(cb, 'Parent');
      | try,
      |     blk = find_system(par, 'LookUnderMasks', 'on', 'RegExp', 'on', 'ReferenceBlock', '^Blocks_lib/CANRxMsgStatus\w*');
      |     msgnam = raptor_get_param_eval(blk{1}, 'msgnam');
      | catch
      |     msgnam = 'MsgName';
      | end
      | 
      | % --- Find Field Name/Units
      | try,
      |     % Name
      |     line_h = get_param(cb, 'LineHandles');
      |     nam = get_param(line_h.Inport(1), 'Name');
      |     nam = strrep(nam, '<', ''); nam = strrep(nam, '>', '');
      |     % Units
      |     units = '';
      |     blk = find_system(par, 'LookUnderMasks', 'on', 'ReferenceBlock', 'Raptor_lib/CAN/raptor_can_rxmsg');
      |     fields = eval(get_param(blk{1}, 'signalInfo'));
      |     fields = fields{1};
      |     for i = 1:length(fields)
      |       fielddata = fields{1,i};
      |       if strcmp(fielddata.Name, nam)
      |           units = fielddata.Units;
      |           break
      |       end
      |     end
      |     nam = strrep(nam, ' ', '');
      | catch,
      |     nam = 'FieldName';
      |     units = 'Units';
      | end
      | if strcmp(custom, 'on')
      |     nam = strrep(custom_nam, '---', nam);
      |     units = strrep(custom_units, '---', units);
      | end
      | 
      | % --- Name Line
      | NameLine([cb '/Out'], 'Inport', nam);
      | 
      | % --- Set Data Types
      | set_param([cb '/Signal Specification'], 'OutDataTypeStr', typ);
      mask Callback custom:
      | raptor_set_param_enable(gcb, 'custom_nam', strcmp(get_param(gcb, 'custom'), 'on'));
      | raptor_set_param_enable(gcb, 'custom_units', strcmp(get_param(gcb, 'custom'), 'on'));
      mask Display:
      | disp(['CAN Rx: Field\n' nam '\n' units ', ' typ]);
      | 
      | port_label('input', 1, 'In');
  CANRxMsgStatus : Blocks_lib/CANRxMsgStatus  samptime=samptime  custom=on  custom_nam='EM2_InvTemp'  msgnam=EM2_InvTemp
  Header : Blocks_lib/Header  width=Landscape  addtext=''
  raptor_can_rxmsg1 : Raptor_lib/CAN/raptor_can_rxmsg  canDefinition=struct('dbcFile', '20220526e_emDrive_NodeID_0x01.dbc','message', 'EM2','comment', '500ms','signals', {{'EM2_InverterBridgeMaxTemp','EM2_MotorSensorTemp'}},'enabled', [ 1 0;],'scaled', [ 1 1;],'canBus', 'bus','messageID', [ 1153;],'idMask', [ 536870911;],'payloadMask', [],'payloadValue', [],'period', [ 0;],'mailbox', '''''','queueSize', [ 1;],'label', [ 1;],'ver', [ 2;],'showID', [ 0;],'showRaw', [ 0;],'fill', [ 0;],'editID', [ 0;],'signalOrder', [ 1;],'signalAscDes', [ 1;])  canBus=bus  mailbox=''  payloadMask=[]  payloadValue=[]  idMask=hex2dec('1FFFFFFF')  queueSize=1  showID=0  label=1  fill=0  id=1153  showRaw=0  showAge=1  signalOrder=1  signalInfo={{struct('Name', 'EM2_InverterBridgeMaxTemp','Startbit', [ 0;],'SignalSize', [ 32;],'ByteOrder', 'LittleEndian','ValueType', 'FLOAT32','Class', 'single','Signed', [ 1;],'Factor', [ 1;],'Offset', [ 0;],'Min', [ -50;],'Max', [ 250;],'Units', 'degC','Comment', 'Ctrl_Bridge_StatusMaxTemp','StartBit', [ 0;]),struct('Name', 'EM2_MotorSensorTemp','Startbit', [ 0;],'SignalSize', [ 32;],'ByteOrder', 'LittleEndian','ValueType', 'FLOAT32','Class', 'single','Signed', [ 1;],'Factor', [ 1;],'Offset', [ 0;],'Min', [ -50;],'Max', [ 250;],'Units', 'degC','Comment', 'Ctrl_Gen_Stat__MotorSensorTemp','StartBit', [ 32;])}}
      settings: SourceProductName=Raptor
  MsgVld : Outport
  Out2 : Outport  Port=2
  wires:
  raptor_can_rxmsg1/2 -> CANRxFieldSingleFloat/1(In)  "EM2_InverterBridgeMaxTemp"
  raptor_can_rxmsg1/1 -> CANRxMsgStatus/2  "Age"
  DiagEnbl/1 -> CANRxMsgStatus/1
  CANRxFieldSingleFloat/1(Out) -> Out2/1
  CANRxMsgStatus/1 -> MsgVld/1

== system VCMGCM1962020b_v2/Fgnd/Sensors/CAN/Inverter/EM2_InvTemp/EM2MtrTemp ==
  DiagEnbl : Inport
  Enable : EnablePort
  CANRxFieldSingleFloat : Subsystem  AncestorBlock=Blocks_lib/CANRxField  mask(CANRxField){typ='double', custom=off, custom_nam='---', custom_units='---'}
      mask prompts: typ "Field Data Type"; custom "Use Custom Name and Units (instead of from .dbc file)"; custom_nam "Custom Name"; custom_units "Custom Units"
      mask help:
      | To be used with the raptor_can_rxmsg block.
      |
      | By default, the field name/units will be inherited from the .dbc file. For Custom Name or Units, check the checkbox. To use the inherited name/units in the custom name/units, use the string '---' to inhereit. For example, to simply add a prefix, the custom name would be something like 'prefix_---'.
      mask init: same as VCMGCM1962020b_v2/Fgnd/Sensors/CAN/Inverter/EM2_InvTemp/EM2InvTemp/CANRxFieldSingleFloat
      mask Callback custom:
      | raptor_set_param_enable(gcb, 'custom_nam', strcmp(get_param(gcb, 'custom'), 'on'));
      | raptor_set_param_enable(gcb, 'custom_units', strcmp(get_param(gcb, 'custom'), 'on'));
      mask Display:
      | disp(['CAN Rx: Field\n' nam '\n' units ', ' typ]);
      | 
      | port_label('input', 1, 'In');
  CANRxMsgStatus : Blocks_lib/CANRxMsgStatus  samptime=samptime  custom=on  custom_nam='EM2_MtrTemp'  msgnam=EM2_MtrTemp
  Header : Blocks_lib/Header  width=Landscape  addtext=''
  raptor_can_rxmsg1 : Raptor_lib/CAN/raptor_can_rxmsg  canDefinition=struct('dbcFile', '20220526e_emDrive_NodeID_0x01.dbc','message', 'EM2','comment', '500ms','signals', {{'EM2_InverterBridgeMaxTemp','EM2_MotorSensorTemp'}},'enabled', [ 0 1;],'scaled', [ 1 1;],'canBus', 'bus','messageID', [ 1153;],'idMask', [ 536870911;],'payloadMask', [],'payloadValue', [],'period', [ 0;],'mailbox', '''''','queueSize', [ 1;],'label', [ 1;],'ver', [ 2;],'showID', [ 0;],'showRaw', [ 0;],'fill', [ 0;],'editID', [ 0;],'signalOrder', [ 1;],'signalAscDes', [ 1;])  canBus=bus  mailbox=''  payloadMask=[]  payloadValue=[]  idMask=hex2dec('1FFFFFFF')  queueSize=1  showID=0  label=1  fill=0  id=1153  showRaw=0  showAge=1  signalOrder=1  signalInfo={{struct('Name', 'EM2_InverterBridgeMaxTemp','Startbit', [ 0;],'SignalSize', [ 32;],'ByteOrder', 'LittleEndian','ValueType', 'FLOAT32','Class', 'single','Signed', [ 1;],'Factor', [ 1;],'Offset', [ 0;],'Min', [ -50;],'Max', [ 250;],'Units', 'degC','Comment', 'Ctrl_Bridge_StatusMaxTemp','StartBit', [ 0;]),struct('Name', 'EM2_MotorSensorTemp','Startbit', [ 0;],'SignalSize', [ 32;],'ByteOrder', 'LittleEndian','ValueType', 'FLOAT32','Class', 'single','Signed', [ 1;],'Factor', [ 1;],'Offset', [ 0;],'Min', [ -50;],'Max', [ 250;],'Units', 'degC','Comment', 'Ctrl_Gen_Stat__MotorSensorTemp','StartBit', [ 32;])}}
      settings: SourceProductName=Raptor
  MsgVld : Outport
  Out2 : Outport  Port=2
  wires:
  raptor_can_rxmsg1/2 -> CANRxFieldSingleFloat/1(In)  "EM2_MotorSensorTemp"
  raptor_can_rxmsg1/1 -> CANRxMsgStatus/2  "Age"
  DiagEnbl/1 -> CANRxMsgStatus/1
  CANRxFieldSingleFloat/1(Out) -> Out2/1
  CANRxMsgStatus/1 -> MsgVld/1

== system VCMGCM1962020b_v2/Fgnd/Sensors/CAN/Inverter/EM3_DCV/EM3DCv ==
  DiagEnbl : Inport
  Enable : EnablePort
  CANRxFieldSingleFloat : Subsystem  AncestorBlock=Blocks_lib/CANRxField  mask(CANRxField){typ='double', custom=off, custom_nam='---', custom_units='---'}
      mask prompts: typ "Field Data Type"; custom "Use Custom Name and Units (instead of from .dbc file)"; custom_nam "Custom Name"; custom_units "Custom Units"
      mask help:
      | To be used with the raptor_can_rxmsg block.
      |
      | By default, the field name/units will be inherited from the .dbc file. For Custom Name or Units, check the checkbox. To use the inherited name/units in the custom name/units, use the string '---' to inhereit. For example, to simply add a prefix, the custom name would be something like 'prefix_---'.
      mask init: same as VCMGCM1962020b_v2/Fgnd/Sensors/CAN/Inverter/EM2_InvTemp/EM2InvTemp/CANRxFieldSingleFloat
      mask Callback custom:
      | raptor_set_param_enable(gcb, 'custom_nam', strcmp(get_param(gcb, 'custom'), 'on'));
      | raptor_set_param_enable(gcb, 'custom_units', strcmp(get_param(gcb, 'custom'), 'on'));
      mask Display:
      | disp(['CAN Rx: Field\n' nam '\n' units ', ' typ]);
      | 
      | port_label('input', 1, 'In');
  CANRxMsgStatus : Blocks_lib/CANRxMsgStatus  samptime=samptime  custom=on  custom_nam='EM3_DCV'  msgnam=EM3_DCV
  Header : Blocks_lib/Header  width=Landscape  addtext=''
  raptor_can_rxmsg1 : Raptor_lib/CAN/raptor_can_rxmsg  canDefinition=struct('dbcFile', '20220526e_emDrive_NodeID_0x01.dbc','message', 'EM3','comment', '40ms','signals', {{'EM3_InverterDcV','EM3_PhaseAmpsRms'}},'enabled', [ 1 0;],'scaled', [ 1 1;],'canBus', 'bus','messageID', [ 897;],'idMask', [ 536870911;],'payloadMask', [],'payloadValue', [],'period', [ 0;],'mailbox', '''''','queueSize', [ 1;],'label', [ 1;],'ver', [ 2;],'showID', [ 0;],'showRaw', [ 0;],'fill', [ 0;],'editID', [ 0;],'signalOrder', [ 1;],'signalAscDes', [ 1;])  canBus=bus  mailbox=''  payloadMask=[]  payloadValue=[]  idMask=hex2dec('1FFFFFFF')  queueSize=1  showID=0  label=1  fill=0  id=897  showRaw=0  showAge=1  signalOrder=1  signalInfo={{struct('Name', 'EM3_InverterDcV','Startbit', [ 0;],'SignalSize', [ 32;],'ByteOrder', 'LittleEndian','ValueType', 'FLOAT32','Class', 'single','Signed', [ 1;],'Factor', [ 1;],'Offset', [ 0;],'Min', [ 0;],'Max', [ 0;],'Units', 'V','Comment', 'HW_Monitor__UDC','StartBit', [ 0;]),struct('Name', 'EM3_PhaseAmpsRms','Startbit', [ 0;],'SignalSize', [ 32;],'ByteOrder', 'LittleEndian','ValueType', 'FLOAT32','Class', 'single','Signed', [ 1;],'Factor', [ 1;],'Offset', [ 0;],'Min', [ 0;],'Max', [ 0;],'Units', 'A','Comment', 'HW_Monitor__Phase_Current','StartBit', [ 32;])}}
      settings: SourceProductName=Raptor
  MsgVld : Outport
  Out2 : Outport  Port=2
  wires:
  raptor_can_rxmsg1/2 -> CANRxFieldSingleFloat/1(In)  "EM3_InverterDcV"
  raptor_can_rxmsg1/1 -> CANRxMsgStatus/2  "Age"
  DiagEnbl/1 -> CANRxMsgStatus/1
  CANRxFieldSingleFloat/1(Out) -> Out2/1
  CANRxMsgStatus/1 -> MsgVld/1
